simulink model "LateralControlTutorial"  (R2021a)
settings: Solver=ode1  StartTime=0.0  StopTime=simStopTime  FixedStep=1e-3  MaxStep=1e-2  MinStep=1e-3  RelTol=5e-3
PostLoadFcn:
  | addpath(fullfile(matlabroot,'toolbox','shared','drivingscenario'));
  | helperLateralControlTutorialSetup
values from neighbouring files (symbols this model uses):
  directions = ones(size(refPoses, 1), 1)    [helperLateralControlTutorialSetup.m]
  speed = 10    [helperCreateDrivingScenario.m]
  speedProfile = ones(size(refPoses, 1), 1)*speed    [helperLateralControlTutorialSetup.m]
  Ts = 0.05    [helperLateralControlTutorialSetup.m]
  wheelbase = 2.8    [helperLateralControlTutorialSetup.m]
undefined symbols (not defined in the file or in its folder): curvatures, refPoses, theta0, x0, y0
libraries: pid_lib x6, simulink_extras x3, drivingvehiclecontroller x2, dspstat3 x1, drivingscenarioandsensors x1, autolibshared x1
settings Model: PacingRate=0.750000  Creator=The MathWorks, Inc.  LastModifiedBy=efrem
settings SolverCC: ZeroCrossAlgorithm=Adaptive  AlgebraicLoopSolver=TrustRegion  DecoupledContinuousIntegration=on  MinimalZcImpactIntegration=on
settings DataIOCC: DSMLogging=off  ReturnWorkspaceOutputs=off
settings DebuggingCC: SFMachineParentedDataDiag=warning  UnderSpecifiedDimensionMsg=warning  ArithmeticOperatorsInVariantConditions=warning
settings SFSimCC: SimUseLocalCustomCode=off  CustomCodeUndefinedFunction=UseInterfaceOnly
settings RTWCC: RTWUseLocalCustomCode=off

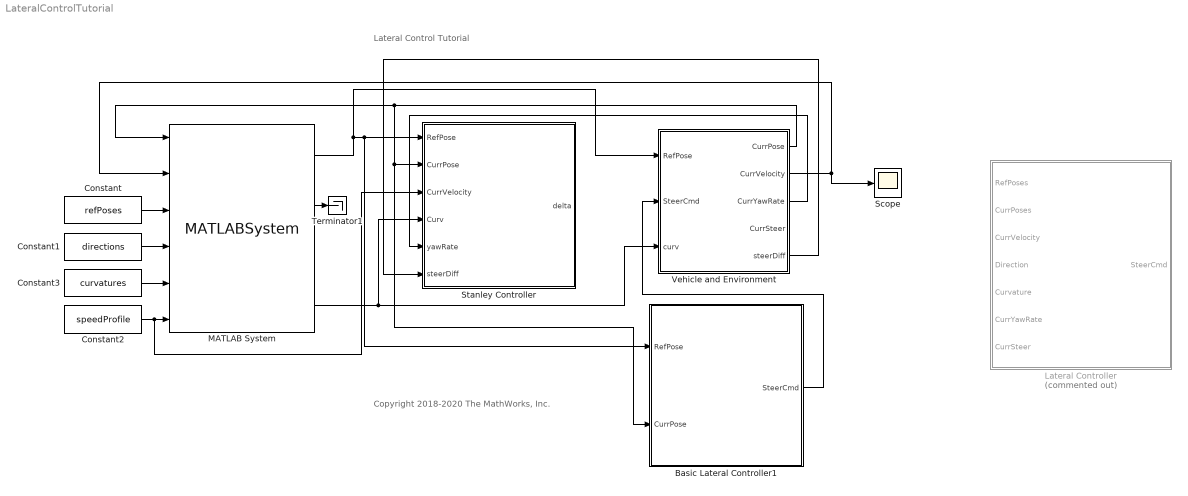
== system LateralControlTutorial ==
  note: Lateral Control Tutorial
  note: Copyright 2018-2020 The MathWorks, Inc.
  Basic Lateral Controller1 : Subsystem
  Constant : Constant  Value=refPoses
  Constant1 : Constant  Value=directions
  Constant2 : Constant  Value=speedProfile
  Constant3 : Constant  Value=curvatures
  Lateral Controller : Subsystem  Commented=on  Variant=on  VariantControlMode=label  VariantControl=Kinematic  LabelModeActiveChoice=Dynamic
  MATLAB System : MATLABSystem  System=HelperPathAnalyzer  Wheelbase=2.8  HasResetOutput=off  SimulateUsing=Interpreted execution
      mask Type: HelperPathAnalyzer
      mask Display:
      | disp(['Helper' char(10) 'Path' char(10) 'Analyzer']);
      | port_label('input',1,'CurrPose');
      | port_label('input',2,'CurrVelocity');
      | port_label('input',3,'RefPoses');
      | port_label('input',4,'Directions');
      | port_label('input',5,'Curvatures');
      | port_label('input',6,'RefVelocities');
      | port_label('output',1,'RefPose');
      | port_label('output',2,'RefVelocity');
      | port_label('output',3,'Direction');
      | port_label('output',4,'Curvature');
  Scope : Scope
  Stanley Controller : Subsystem
  Terminator1 : Terminator
  Vehicle and Environment : Subsystem
  wires:
  Constant/1 -> MATLAB System/3
  MATLAB System/2 -> Terminator1/1
  Constant1/1 -> MATLAB System/4
  Vehicle and Environment/1(CurrPose) -> Basic Lateral Controller1/2(CurrPose), Stanley Controller/2(CurrPose), MATLAB System/1
  Vehicle and Environment/2(CurrVelocity) -> Scope/1, MATLAB System/2
  MATLAB System/1 -> Basic Lateral Controller1/1(RefPose), Stanley Controller/1(RefPose), Vehicle and Environment/1(RefPose)
  MATLAB System/4 -> Stanley Controller/4(Curv), Vehicle and Environment/3(curv)
  Constant3/1 -> MATLAB System/5
  Constant2/1 -> Stanley Controller/3(CurrVelocity), MATLAB System/6
  Basic Lateral Controller1/1(SteerCmd) -> Vehicle and Environment/2(SteerCmd)
  Vehicle and Environment/3(CurrYawRate) -> Stanley Controller/5(yawRate)
  Vehicle and Environment/5(steerDiff) -> Stanley Controller/6(steerDiff)

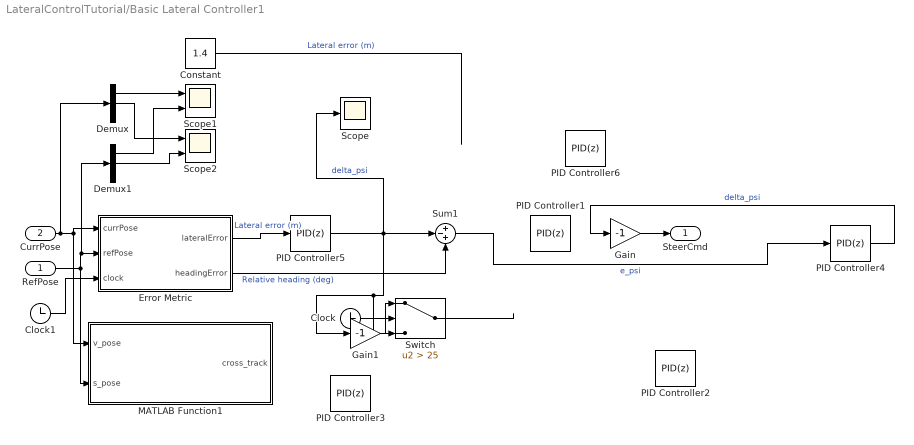
== system LateralControlTutorial/Basic Lateral Controller1 ==
  RefPose : Inport
  CurrPose : Inport  Port=2
  Clock : Clock
  Clock1 : Clock
  Constant : Constant  Value=1.4
  Demux : Demux  Outputs=3
  Demux1 : Demux  Outputs=3
  Error Metric : MATLAB Function  TreatAsAtomicUnit=on  mask{wheelbase=wheelbase}
      mask prompts: wheelbase "Wheelbase of vehicle"
  Gain : Gain  Gain=-1
  Gain1 : Gain  Gain=-1
  MATLAB Function1 : MATLAB Function  TreatAsAtomicUnit=on
  PID Controller1 : pid_lib/PID Controller  Controller=PID  Form=Parallel  TimeDomain=Discrete-time  UseExternalTs=off  SampleTime=-1  IntegratorMethod=Forward Euler  FilterMethod=Forward Euler  ControllerParametersSource=internal  P=0.67  I=0.12  D=0.32  UseFilter=on  N=100  TunerSelectOption=Transfer Function Based (PID Tuner App)  InitialConditionSource=internal  InitialConditionForIntegrator=0  InitialConditionForFilter=0  DifferentiatorICPrevScaledInput=0  ExternalReset=none  TrackingMode=off  Kt=1  LimitOutput=on  SatLimitsSource=internal  UpperSaturationLimit=45  LowerSaturationLimit=-45  LinearizeAsGain=on  AntiWindupMode=none  Kb=1  POutMin=[]  POutMax=[]  IOutMin=[]  IOutMax=[]  DOutMin=[]  DOutMax=[]  NOutMin=[]  NOutMax=[]  SumOutMin=[]  SumOutMax=[]  SaturationOutMin=[]  SaturationOutMax=[]  PParamMin=[]  PParamMax=[]  IParamMin=[]  IParamMax=[]  DParamMin=[]  DParamMax=[]  NParamMin=[]  NParamMax=[]  KbParamMin=[]  KbParamMax=[]  KtParamMin=[]  KtParamMax=[]  KbOutMin=[]  KbOutMax=[]  KtOutMin=[]  KtOutMax=[]  IntegratorOutMin=[]  IntegratorOutMax=[]  FilterOutMin=[]  FilterOutMax=[]  SumI1OutMin=[]  SumI1OutMax=[]  SumI2OutMin=[]  SumI2OutMax=[]  SumI3OutMin=[]  SumI3OutMax=[]  SumI4OutMin=[]  SumI4OutMax=[]  SumDOutMin=[]  SumDOutMax=[]  DifferentiatorOutMin=[]  DifferentiatorOutMax=[]  FilterDiffOutCoefMin=[]  FilterDiffOutCoefMax=[]  ReciprocalOutMin=[]  ReciprocalOutMax=[]  SumDenOutMin=[]  SumDenOutMax=[]  SumNumOutMin=[]  SumNumOutMax=[]  DivideOutMin=[]  DivideOutMax=[]  UdiffTsProdOutMin=[]  UdiffTsProdOutMax=[]  NTsProdOutMin=[]  NTsProdOutMax=[]  UintegralTsProdOutMin=[]  UintegralTsProdOutMax=[]  UngainTsProdOutMin=[]  UngainTsProdOutMax=[]  IntegratorContinuousStateAttributes=''  IntegratorStateMustResolveToSignalObject=off  IntegratorRTWStateStorageClass=Auto  FilterContinuousStateAttributes=''  FilterStateMustResolveToSignalObject=off  FilterRTWStateStorageClass=Auto  ParallelPVariant=InternalParameters  IdealPVariant=Disabled  IVariant=InternalParameters  DVariant=InternalParameters  IntegratorVariant=Discrete  SatVariant=Enabled  AWVariant=Passthrough  PCopyVariant=Disabled  TRVariant=Disabled  FdbkBlocksVariant=Forward  IdealPFdbkVariant=Disabled  SatFdbkVariant=Disabled  DerivativeFilterVariant=ForwardEulerFilter  NVariant=InternalParameters  NCopyVariant=Disabled  FilterICVariant=InternalICsFilter  IntegratorICVariant=InternalICs  ExternalResetVariant=Disabled  TRSumVariant=Passthrough  SumFdbkVariant=Disabled  SumVariant=Sum_PID  TsampFilterVariant=InternalTs  TsampNgainVariant=Passthrough  TsampIntegralVariant=Passthrough  ExternalSaturationOutDataTypeStr=Inherit: Same as second input
  PID Controller2 : pid_lib/PID Controller  Controller=PID  Form=Parallel  TimeDomain=Discrete-time  UseExternalTs=off  SampleTime=-1  IntegratorMethod=Forward Euler  FilterMethod=Forward Euler  ControllerParametersSource=internal  P=1.5  I=0.4  D=0.4  UseFilter=on  N=1000  TunerSelectOption=Transfer Function Based (PID Tuner App)  InitialConditionSource=internal  InitialConditionForIntegrator=0  InitialConditionForFilter=0  DifferentiatorICPrevScaledInput=0  ExternalReset=none  TrackingMode=off  Kt=1  LimitOutput=on  SatLimitsSource=internal  UpperSaturationLimit=45  LowerSaturationLimit=-45  LinearizeAsGain=on  AntiWindupMode=none  Kb=1  POutMin=[]  POutMax=[]  IOutMin=[]  IOutMax=[]  DOutMin=[]  DOutMax=[]  NOutMin=[]  NOutMax=[]  SumOutMin=[]  SumOutMax=[]  SaturationOutMin=[]  SaturationOutMax=[]  PParamMin=[]  PParamMax=[]  IParamMin=[]  IParamMax=[]  DParamMin=[]  DParamMax=[]  NParamMin=[]  NParamMax=[]  KbParamMin=[]  KbParamMax=[]  KtParamMin=[]  KtParamMax=[]  KbOutMin=[]  KbOutMax=[]  KtOutMin=[]  KtOutMax=[]  IntegratorOutMin=[]  IntegratorOutMax=[]  FilterOutMin=[]  FilterOutMax=[]  SumI1OutMin=[]  SumI1OutMax=[]  SumI2OutMin=[]  SumI2OutMax=[]  SumI3OutMin=[]  SumI3OutMax=[]  SumI4OutMin=[]  SumI4OutMax=[]  SumDOutMin=[]  SumDOutMax=[]  DifferentiatorOutMin=[]  DifferentiatorOutMax=[]  FilterDiffOutCoefMin=[]  FilterDiffOutCoefMax=[]  ReciprocalOutMin=[]  ReciprocalOutMax=[]  SumDenOutMin=[]  SumDenOutMax=[]  SumNumOutMin=[]  SumNumOutMax=[]  DivideOutMin=[]  DivideOutMax=[]  UdiffTsProdOutMin=[]  UdiffTsProdOutMax=[]  NTsProdOutMin=[]  NTsProdOutMax=[]  UintegralTsProdOutMin=[]  UintegralTsProdOutMax=[]  UngainTsProdOutMin=[]  UngainTsProdOutMax=[]  IntegratorContinuousStateAttributes=''  IntegratorStateMustResolveToSignalObject=off  IntegratorRTWStateStorageClass=Auto  FilterContinuousStateAttributes=''  FilterStateMustResolveToSignalObject=off  FilterRTWStateStorageClass=Auto  ParallelPVariant=InternalParameters  IdealPVariant=Disabled  IVariant=InternalParameters  DVariant=InternalParameters  IntegratorVariant=Discrete  SatVariant=Enabled  AWVariant=Passthrough  PCopyVariant=Disabled  TRVariant=Disabled  FdbkBlocksVariant=Forward  IdealPFdbkVariant=Disabled  SatFdbkVariant=Disabled  DerivativeFilterVariant=ForwardEulerFilter  NVariant=InternalParameters  NCopyVariant=Disabled  FilterICVariant=InternalICsFilter  IntegratorICVariant=InternalICs  ExternalResetVariant=Disabled  TRSumVariant=Passthrough  SumFdbkVariant=Disabled  SumVariant=Sum_PID  TsampFilterVariant=InternalTs  TsampNgainVariant=Passthrough  TsampIntegralVariant=Passthrough  ExternalSaturationOutDataTypeStr=Inherit: Same as second input
  PID Controller3 : pid_lib/PID Controller  Controller=PID  Form=Parallel  TimeDomain=Discrete-time  UseExternalTs=off  SampleTime=-1  IntegratorMethod=Forward Euler  FilterMethod=Forward Euler  ControllerParametersSource=internal  P=0.4  I=0  D=0  UseFilter=on  N=100  TunerSelectOption=Transfer Function Based (PID Tuner App)  InitialConditionSource=internal  InitialConditionForIntegrator=0  InitialConditionForFilter=0  DifferentiatorICPrevScaledInput=0  ExternalReset=none  TrackingMode=off  Kt=1  LimitOutput=off  SatLimitsSource=internal  UpperSaturationLimit=0.5  LowerSaturationLimit=-0.5  LinearizeAsGain=on  AntiWindupMode=none  Kb=1  POutMin=[]  POutMax=[]  IOutMin=[]  IOutMax=[]  DOutMin=[]  DOutMax=[]  NOutMin=[]  NOutMax=[]  SumOutMin=[]  SumOutMax=[]  SaturationOutMin=[]  SaturationOutMax=[]  PParamMin=[]  PParamMax=[]  IParamMin=[]  IParamMax=[]  DParamMin=[]  DParamMax=[]  NParamMin=[]  NParamMax=[]  KbParamMin=[]  KbParamMax=[]  KtParamMin=[]  KtParamMax=[]  KbOutMin=[]  KbOutMax=[]  KtOutMin=[]  KtOutMax=[]  IntegratorOutMin=[]  IntegratorOutMax=[]  FilterOutMin=[]  FilterOutMax=[]  SumI1OutMin=[]  SumI1OutMax=[]  SumI2OutMin=[]  SumI2OutMax=[]  SumI3OutMin=[]  SumI3OutMax=[]  SumI4OutMin=[]  SumI4OutMax=[]  SumDOutMin=[]  SumDOutMax=[]  DifferentiatorOutMin=[]  DifferentiatorOutMax=[]  FilterDiffOutCoefMin=[]  FilterDiffOutCoefMax=[]  ReciprocalOutMin=[]  ReciprocalOutMax=[]  SumDenOutMin=[]  SumDenOutMax=[]  SumNumOutMin=[]  SumNumOutMax=[]  DivideOutMin=[]  DivideOutMax=[]  UdiffTsProdOutMin=[]  UdiffTsProdOutMax=[]  NTsProdOutMin=[]  NTsProdOutMax=[]  UintegralTsProdOutMin=[]  UintegralTsProdOutMax=[]  UngainTsProdOutMin=[]  UngainTsProdOutMax=[]  IntegratorContinuousStateAttributes=''  IntegratorStateMustResolveToSignalObject=off  IntegratorRTWStateStorageClass=Auto  FilterContinuousStateAttributes=''  FilterStateMustResolveToSignalObject=off  FilterRTWStateStorageClass=Auto  ParallelPVariant=InternalParameters  IdealPVariant=Disabled  IVariant=InternalParameters  DVariant=InternalParameters  IntegratorVariant=Discrete  SatVariant=Disabled  AWVariant=Passthrough  PCopyVariant=Disabled  TRVariant=Disabled  FdbkBlocksVariant=Forward  IdealPFdbkVariant=Disabled  SatFdbkVariant=Disabled  DerivativeFilterVariant=ForwardEulerFilter  NVariant=InternalParameters  NCopyVariant=Disabled  FilterICVariant=InternalICsFilter  IntegratorICVariant=InternalICs  ExternalResetVariant=Disabled  TRSumVariant=Passthrough  SumFdbkVariant=Disabled  SumVariant=Sum_PID  TsampFilterVariant=InternalTs  TsampNgainVariant=Passthrough  TsampIntegralVariant=Passthrough  ExternalSaturationOutDataTypeStr=Inherit: Same as second input
  PID Controller4 : pid_lib/PID Controller  Controller=PID  Form=Parallel  TimeDomain=Discrete-time  UseExternalTs=off  SampleTime=-1  IntegratorMethod=Forward Euler  FilterMethod=Forward Euler  ControllerParametersSource=internal  P=1.5  I=0.4  D=0.4  UseFilter=on  N=600  TunerSelectOption=Transfer Function Based (PID Tuner App)  InitialConditionSource=internal  InitialConditionForIntegrator=0  InitialConditionForFilter=0  DifferentiatorICPrevScaledInput=0  ExternalReset=none  TrackingMode=off  Kt=1  LimitOutput=on  SatLimitsSource=internal  UpperSaturationLimit=45  LowerSaturationLimit=-45  LinearizeAsGain=on  AntiWindupMode=none  Kb=1  POutMin=[]  POutMax=[]  IOutMin=[]  IOutMax=[]  DOutMin=[]  DOutMax=[]  NOutMin=[]  NOutMax=[]  SumOutMin=[]  SumOutMax=[]  SaturationOutMin=[]  SaturationOutMax=[]  PParamMin=[]  PParamMax=[]  IParamMin=[]  IParamMax=[]  DParamMin=[]  DParamMax=[]  NParamMin=[]  NParamMax=[]  KbParamMin=[]  KbParamMax=[]  KtParamMin=[]  KtParamMax=[]  KbOutMin=[]  KbOutMax=[]  KtOutMin=[]  KtOutMax=[]  IntegratorOutMin=[]  IntegratorOutMax=[]  FilterOutMin=[]  FilterOutMax=[]  SumI1OutMin=[]  SumI1OutMax=[]  SumI2OutMin=[]  SumI2OutMax=[]  SumI3OutMin=[]  SumI3OutMax=[]  SumI4OutMin=[]  SumI4OutMax=[]  SumDOutMin=[]  SumDOutMax=[]  DifferentiatorOutMin=[]  DifferentiatorOutMax=[]  FilterDiffOutCoefMin=[]  FilterDiffOutCoefMax=[]  ReciprocalOutMin=[]  ReciprocalOutMax=[]  SumDenOutMin=[]  SumDenOutMax=[]  SumNumOutMin=[]  SumNumOutMax=[]  DivideOutMin=[]  DivideOutMax=[]  UdiffTsProdOutMin=[]  UdiffTsProdOutMax=[]  NTsProdOutMin=[]  NTsProdOutMax=[]  UintegralTsProdOutMin=[]  UintegralTsProdOutMax=[]  UngainTsProdOutMin=[]  UngainTsProdOutMax=[]  IntegratorContinuousStateAttributes=''  IntegratorStateMustResolveToSignalObject=off  IntegratorRTWStateStorageClass=Auto  FilterContinuousStateAttributes=''  FilterStateMustResolveToSignalObject=off  FilterRTWStateStorageClass=Auto  ParallelPVariant=InternalParameters  IdealPVariant=Disabled  IVariant=InternalParameters  DVariant=InternalParameters  IntegratorVariant=Discrete  SatVariant=Enabled  AWVariant=Passthrough  PCopyVariant=Disabled  TRVariant=Disabled  FdbkBlocksVariant=Forward  IdealPFdbkVariant=Disabled  SatFdbkVariant=Disabled  DerivativeFilterVariant=ForwardEulerFilter  NVariant=InternalParameters  NCopyVariant=Disabled  FilterICVariant=InternalICsFilter  IntegratorICVariant=InternalICs  ExternalResetVariant=Disabled  TRSumVariant=Passthrough  SumFdbkVariant=Disabled  SumVariant=Sum_PID  TsampFilterVariant=InternalTs  TsampNgainVariant=Passthrough  TsampIntegralVariant=Passthrough  ExternalSaturationOutDataTypeStr=Inherit: Same as second input
  PID Controller5 : pid_lib/PID Controller  Controller=PID  Form=Parallel  TimeDomain=Discrete-time  UseExternalTs=off  SampleTime=-1  IntegratorMethod=Forward Euler  FilterMethod=Forward Euler  ControllerParametersSource=internal  P=8  I=2  D=0  UseFilter=on  N=100  TunerSelectOption=Transfer Function Based (PID Tuner App)  InitialConditionSource=internal  InitialConditionForIntegrator=0  InitialConditionForFilter=0  DifferentiatorICPrevScaledInput=0  ExternalReset=none  TrackingMode=off  Kt=1  LimitOutput=off  SatLimitsSource=internal  UpperSaturationLimit=0.5  LowerSaturationLimit=-0.5  LinearizeAsGain=on  AntiWindupMode=none  Kb=1  POutMin=[]  POutMax=[]  IOutMin=[]  IOutMax=[]  DOutMin=[]  DOutMax=[]  NOutMin=[]  NOutMax=[]  SumOutMin=[]  SumOutMax=[]  SaturationOutMin=[]  SaturationOutMax=[]  PParamMin=[]  PParamMax=[]  IParamMin=[]  IParamMax=[]  DParamMin=[]  DParamMax=[]  NParamMin=[]  NParamMax=[]  KbParamMin=[]  KbParamMax=[]  KtParamMin=[]  KtParamMax=[]  KbOutMin=[]  KbOutMax=[]  KtOutMin=[]  KtOutMax=[]  IntegratorOutMin=[]  IntegratorOutMax=[]  FilterOutMin=[]  FilterOutMax=[]  SumI1OutMin=[]  SumI1OutMax=[]  SumI2OutMin=[]  SumI2OutMax=[]  SumI3OutMin=[]  SumI3OutMax=[]  SumI4OutMin=[]  SumI4OutMax=[]  SumDOutMin=[]  SumDOutMax=[]  DifferentiatorOutMin=[]  DifferentiatorOutMax=[]  FilterDiffOutCoefMin=[]  FilterDiffOutCoefMax=[]  ReciprocalOutMin=[]  ReciprocalOutMax=[]  SumDenOutMin=[]  SumDenOutMax=[]  SumNumOutMin=[]  SumNumOutMax=[]  DivideOutMin=[]  DivideOutMax=[]  UdiffTsProdOutMin=[]  UdiffTsProdOutMax=[]  NTsProdOutMin=[]  NTsProdOutMax=[]  UintegralTsProdOutMin=[]  UintegralTsProdOutMax=[]  UngainTsProdOutMin=[]  UngainTsProdOutMax=[]  IntegratorContinuousStateAttributes=''  IntegratorStateMustResolveToSignalObject=off  IntegratorRTWStateStorageClass=Auto  FilterContinuousStateAttributes=''  FilterStateMustResolveToSignalObject=off  FilterRTWStateStorageClass=Auto  ParallelPVariant=InternalParameters  IdealPVariant=Disabled  IVariant=InternalParameters  DVariant=InternalParameters  IntegratorVariant=Discrete  SatVariant=Disabled  AWVariant=Passthrough  PCopyVariant=Disabled  TRVariant=Disabled  FdbkBlocksVariant=Forward  IdealPFdbkVariant=Disabled  SatFdbkVariant=Disabled  DerivativeFilterVariant=ForwardEulerFilter  NVariant=InternalParameters  NCopyVariant=Disabled  FilterICVariant=InternalICsFilter  IntegratorICVariant=InternalICs  ExternalResetVariant=Disabled  TRSumVariant=Passthrough  SumFdbkVariant=Disabled  SumVariant=Sum_PID  TsampFilterVariant=InternalTs  TsampNgainVariant=Passthrough  TsampIntegralVariant=Passthrough  ExternalSaturationOutDataTypeStr=Inherit: Same as second input
  PID Controller6 : pid_lib/PID Controller  Controller=PID  Form=Parallel  TimeDomain=Discrete-time  UseExternalTs=off  SampleTime=-1  IntegratorMethod=Forward Euler  FilterMethod=Forward Euler  ControllerParametersSource=internal  P=2  I=0.02  D=0  UseFilter=on  N=100  TunerSelectOption=Transfer Function Based (PID Tuner App)  InitialConditionSource=internal  InitialConditionForIntegrator=0  InitialConditionForFilter=0  DifferentiatorICPrevScaledInput=0  ExternalReset=none  TrackingMode=off  Kt=1  LimitOutput=off  SatLimitsSource=internal  UpperSaturationLimit=0.5  LowerSaturationLimit=-0.5  LinearizeAsGain=on  AntiWindupMode=none  Kb=1  POutMin=[]  POutMax=[]  IOutMin=[]  IOutMax=[]  DOutMin=[]  DOutMax=[]  NOutMin=[]  NOutMax=[]  SumOutMin=[]  SumOutMax=[]  SaturationOutMin=[]  SaturationOutMax=[]  PParamMin=[]  PParamMax=[]  IParamMin=[]  IParamMax=[]  DParamMin=[]  DParamMax=[]  NParamMin=[]  NParamMax=[]  KbParamMin=[]  KbParamMax=[]  KtParamMin=[]  KtParamMax=[]  KbOutMin=[]  KbOutMax=[]  KtOutMin=[]  KtOutMax=[]  IntegratorOutMin=[]  IntegratorOutMax=[]  FilterOutMin=[]  FilterOutMax=[]  SumI1OutMin=[]  SumI1OutMax=[]  SumI2OutMin=[]  SumI2OutMax=[]  SumI3OutMin=[]  SumI3OutMax=[]  SumI4OutMin=[]  SumI4OutMax=[]  SumDOutMin=[]  SumDOutMax=[]  DifferentiatorOutMin=[]  DifferentiatorOutMax=[]  FilterDiffOutCoefMin=[]  FilterDiffOutCoefMax=[]  ReciprocalOutMin=[]  ReciprocalOutMax=[]  SumDenOutMin=[]  SumDenOutMax=[]  SumNumOutMin=[]  SumNumOutMax=[]  DivideOutMin=[]  DivideOutMax=[]  UdiffTsProdOutMin=[]  UdiffTsProdOutMax=[]  NTsProdOutMin=[]  NTsProdOutMax=[]  UintegralTsProdOutMin=[]  UintegralTsProdOutMax=[]  UngainTsProdOutMin=[]  UngainTsProdOutMax=[]  IntegratorContinuousStateAttributes=''  IntegratorStateMustResolveToSignalObject=off  IntegratorRTWStateStorageClass=Auto  FilterContinuousStateAttributes=''  FilterStateMustResolveToSignalObject=off  FilterRTWStateStorageClass=Auto  ParallelPVariant=InternalParameters  IdealPVariant=Disabled  IVariant=InternalParameters  DVariant=InternalParameters  IntegratorVariant=Discrete  SatVariant=Disabled  AWVariant=Passthrough  PCopyVariant=Disabled  TRVariant=Disabled  FdbkBlocksVariant=Forward  IdealPFdbkVariant=Disabled  SatFdbkVariant=Disabled  DerivativeFilterVariant=ForwardEulerFilter  NVariant=InternalParameters  NCopyVariant=Disabled  FilterICVariant=InternalICsFilter  IntegratorICVariant=InternalICs  ExternalResetVariant=Disabled  TRSumVariant=Passthrough  SumFdbkVariant=Disabled  SumVariant=Sum_PID  TsampFilterVariant=InternalTs  TsampNgainVariant=Passthrough  TsampIntegralVariant=Passthrough  ExternalSaturationOutDataTypeStr=Inherit: Same as second input
  Scope : Scope
  Scope1 : Scope  NumInputPorts=2
  Scope2 : Scope  NumInputPorts=2
  Sum1 : Sum  Inputs=+-+
  Switch : Switch  Criteria=u2 > Threshold  Threshold=25
  SteerCmd : Outport
  wires:
  PID Controller5/1 -> Sum1/2, Switch/3, Gain1/1, Scope/1  "delta_psi"
  Sum1/1 -> PID Controller4/1  "e_psi"
  PID Controller4/1 -> Gain/1  "delta_psi"
  CurrPose/1 -> Demux/1, MATLAB Function1/1(v_pose), Error Metric/1(currPose)
  RefPose/1 -> MATLAB Function1/2(s_pose), Demux1/1, Error Metric/2(refPose)
  Error Metric/1(lateralError) -> PID Controller5/1  "Lateral error (m)"
  Error Metric/2(headingError) -> Sum1/3  "Relative heading (deg)"
  Gain/1 -> SteerCmd/1
  Constant/1 -> ?  "Lateral error (m)"
  Clock/1 -> Switch/2
  Gain1/1 -> Switch/1
  Clock1/1 -> Error Metric/3(clock)
  Demux/1 -> Scope1/1
  Demux1/1 -> Scope1/2
  Demux/2 -> Scope2/1
  Demux1/2 -> Scope2/2
  Switch/1 -> ?

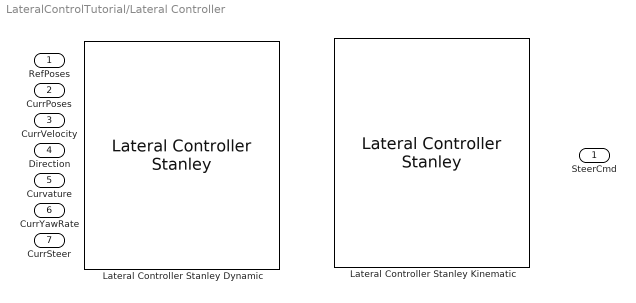
== system LateralControlTutorial/Lateral Controller ==
  "RefPoses " : Inport
  "CurrPoses " : Inport  Port=2
  "CurrVelocity " : Inport  Port=3
  "Direction " : Inport  Port=4
  "Curvature " : Inport  Port=5
  "CurrYawRate " : Inport  Port=6
  "CurrSteer " : Inport  Port=7
  Lateral Controller Stanley Dynamic : drivingvehiclecontroller/Lateral Controller Stanley  VariantControl=Dynamic  ModelType=Dynamic bicycle model  PositionGainF=2.5  PositionGainR=2.5  YawRateGain=0.5  DelayGain=0.2  VehicleMass=1575  Lf=1.2  Lr=1.6  TireStiffness=19000  Wheelbase=wheelbase  MaxSteeringAngle=35
      settings: SourceProductBaseCode=DR
  Lateral Controller Stanley Kinematic : drivingvehiclecontroller/Lateral Controller Stanley  VariantControl=Kinematic  ModelType=Kinematic bicycle model  PositionGainF=2.5  PositionGainR=2.5  YawRateGain=0.2  DelayGain=0.2  VehicleMass=1575  Lf=1.2  Lr=1.6  TireStiffness=19000  Wheelbase=wheelbase  MaxSteeringAngle=35
      settings: SourceProductBaseCode=DR
  " SteerCmd" : Outport  VectorParamsAs1DForOutWhenUnconnected=off

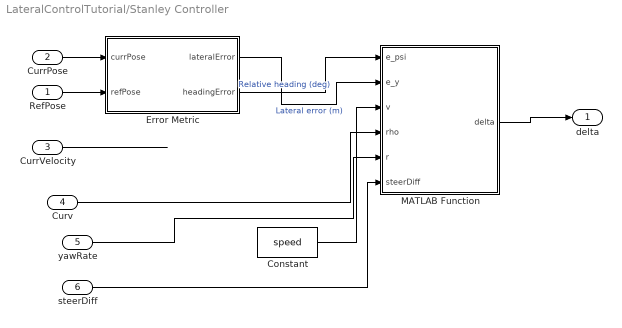
== system LateralControlTutorial/Stanley Controller ==
  RefPose : Inport
  CurrPose : Inport  Port=2
  CurrVelocity : Inport  Port=3
  Curv : Inport  Port=4
  yawRate : Inport  Port=5
  steerDiff : Inport  Port=6
  Constant : Constant  Value=speed
  Error Metric : MATLAB Function  TreatAsAtomicUnit=on  mask{wheelbase=wheelbase}
      mask prompts: wheelbase "Wheelbase of vehicle"
  MATLAB Function : MATLAB Function  TreatAsAtomicUnit=on
  delta : Outport
  wires:
  CurrPose/1 -> Error Metric/1(currPose)
  RefPose/1 -> Error Metric/2(refPose)
  Error Metric/1(lateralError) -> MATLAB Function/2(e_y)  "Lateral error (m)"
  Error Metric/2(headingError) -> MATLAB Function/1(e_psi)  "Relative heading (deg)"
  CurrVelocity/1 -> ?
  Curv/1 -> MATLAB Function/4(rho)
  yawRate/1 -> MATLAB Function/5(r)
  MATLAB Function/1(delta) -> delta/1
  Constant/1 -> MATLAB Function/3(v)
  steerDiff/1 -> MATLAB Function/6(steerDiff)

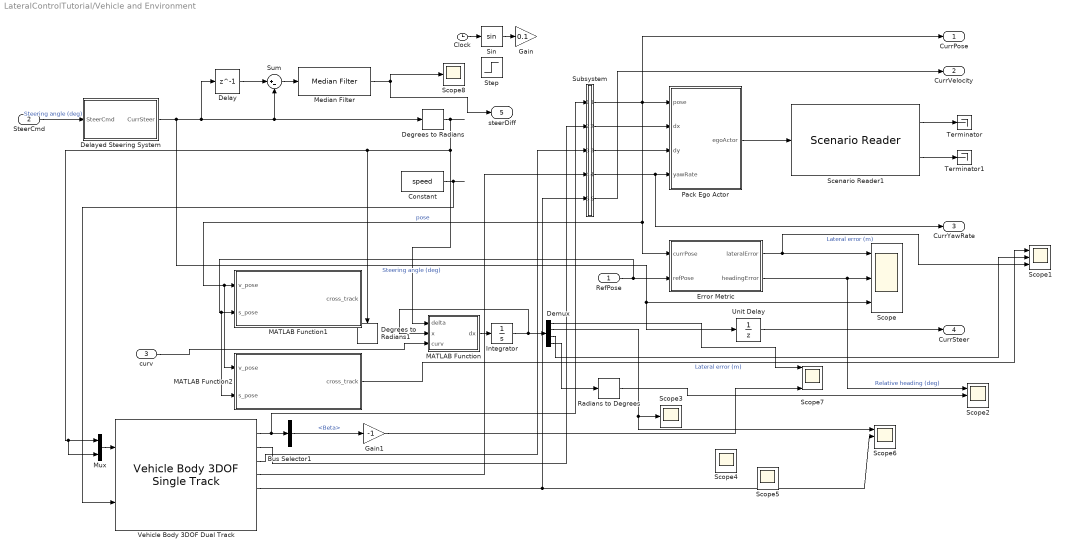
== system LateralControlTutorial/Vehicle and Environment ==
  RefPose : Inport
  SteerCmd : Inport  Port=2
  curv : Inport  Port=3
  Bus Selector1 : BusSelector  OutputSignals=BdyFrm.Cg.Ang.Beta
  Clock : Clock
  Constant : Constant  Value=speed
  Degrees to Radians : simulink_extras/Transformations/Degrees to Radians
  Degrees to Radians1 : simulink_extras/Transformations/Degrees to Radians
  Delay : Delay  DelayLength=1
  Delayed Steering System : Subsystem
  Demux : Demux
  Error Metric : MATLAB Function  TreatAsAtomicUnit=on  mask{wheelbase=wheelbase}
      mask prompts: wheelbase "Wheelbase of vehicle"
  Gain : Gain  Gain=0.1
  Gain1 : Gain  Gain=-1
  Integrator : Integrator  InitialCondition=[0; 0;0;0]
  MATLAB Function : MATLAB Function  TreatAsAtomicUnit=on
  MATLAB Function1 : MATLAB Function  TreatAsAtomicUnit=on
  MATLAB Function2 : MATLAB Function  TreatAsAtomicUnit=on
  Median Filter : dspstat3/Median Filter  WindowLength=10  SimulateUsing=Interpreted execution
      settings: SourceProductBaseCode=DS
  Mux : Mux  Inputs=2
  Pack Ego Actor : MATLAB Function  TreatAsAtomicUnit=on
  Radians to Degrees : simulink_extras/Transformations/Radians to Degrees
  Scenario Reader1 : drivingscenarioandsensors/Scenario Reader  ScenarioSource=From file  ScenarioFileName=LateralControl.mat  ScenarioVariableName=scenario  OutputCoordinateSystem=Vehicle coordinates  EgoVehicleSource=Input port  EgoVehicleActorID=1  OrientVehiclesOnRoad=off  OutputEgoVehiclePose=off  SampleTime=Ts  LaneBoundaryOutput=Ego vehicle lane boundaries  LaneBoundaryDistance=0:0.5:9.5  LaneBoundaryLocation=Center of lane markings  BusNameSource=Property  BusName=BusActors  BusNumActorsSource=Scenario  BusNumActors=100  BusName2Source=Auto  BusName2=BusLaneBoundaries  BusNumLaneBoundariesSource=Scenario  BusNumLaneBoundaries=10  BusName3Source=Auto  BusName3=BusEgoActor  ShowCoordinateLabels=on  SimulateUsing=Interpreted execution
  Scope{,1..2,6} (4 alike) : Scope  NumInputPorts=3
  Scope{3..5,8} (4 alike) : Scope
  Scope7 : Scope  NumInputPorts=4
  Sin : Trigonometry
  Step : Step  Time=0  After=-0.2  SampleTime=0
  Subsystem : Subsystem
  Sum : Sum  Inputs=|+-
  Terminator : Terminator
  Terminator1 : Terminator
  Unit Delay : UnitDelay  SampleTime=0.05  HasFrameUpgradeWarning=on
  Vehicle Body 3DOF Dual Track : autolibshared/Vehicle Body 3DOF Single Track  trackMode=Dual  inputMode=External longitudinal velocity  frontSteerMode=on  rearSteerMode=off  windMode=off  muMode=off  extFMode=off  extMMode=off  htchFMode=off  htchMMode=off  extXo=off  extpsio=off  extxdoto=off  extro=off  extYo=off  extTamb=off  extydoto=off  aMode=2  NF=2  NR=2  m=2000  a=1.4  b=1.6  h=0.35  dh=1  hh=0.2  X_o=0  xdot_o=0  CalphaMode=off  sigmaMode=on  d=0  hl=0  w=[1.4,1.4]  Cy_f=12e3  Cy_r=11e3  sigma_f=.1  sigma_r=.1  alpha_f_brk=[-.1 .1]  Cy_f_data=[-9e3 9e3]  alpha_r_brk=[-.1 .1]  Cy_r_data=[-9e3 9e3]  Y_o=0  ydot_o=0  Izz=4000  psi_o=0  r_o=0  Af=2  Cd=.3  Cl=.1  Cpm=.1  beta_w=[0:0.01:0.3]  Cs=[0:0.03:0.9]  Cym=[0:0.01:0.3]  Pabs=101325  Tair=273  g=9.81  mu=1  xdot_tol=.01  Fznom=5000  Fxtire_sat=7e4  Fytire_sat=7e4  longOff=0  latOff=0  vertOff=0  wrapAng=off
      settings: SourceProductBaseCode=PW,DR,MT,UV,VE
  CurrPose : Outport  VectorParamsAs1DForOutWhenUnconnected=off
  CurrVelocity : Outport  Port=2  VectorParamsAs1DForOutWhenUnconnected=off
  CurrYawRate : Outport  Port=3  VectorParamsAs1DForOutWhenUnconnected=off
  CurrSteer : Outport  Port=4  VectorParamsAs1DForOutWhenUnconnected=off
  steerDiff : Outport  Port=5
  wires:
  Subsystem/2(dx) -> Pack Ego Actor/2(dx)
  Subsystem/4(CurrYawRate) -> CurrYawRate/1, Pack Ego Actor/4(yawRate)
  Subsystem/3(dy) -> Pack Ego Actor/3(dy)
  Subsystem/1(CurrPose) -> CurrPose/1, Pack Ego Actor/1(pose), Error Metric/1(currPose), MATLAB Function2/1(v_pose), MATLAB Function1/1(v_pose)  "pose"
  Error Metric/1(lateralError) -> Scope1/3, Scope/1  "Lateral error (m)"
  RefPose/1 -> MATLAB Function2/2(s_pose), MATLAB Function1/2(s_pose), Error Metric/2(refPose)
  Error Metric/2(headingError) -> Scope2/1, Scope/2  "Relative heading (deg)"
  Degrees to Radians/1 -> Mux/2, Mux/1, Degrees to Radians1/1, MATLAB Function/1(delta)
  Constant/1 -> Vehicle Body 3DOF Dual Track/2
  Delayed Steering System/1(CurrSteer) -> Delay/1, Sum/2, Degrees to Radians/1, Unit Delay/1, Scope/3  "Steering angle (deg)"
  Unit Delay/1 -> CurrSteer/1
  Scenario Reader1/1 -> Terminator/1
  Subsystem/5(CurrVelocity) -> CurrVelocity/1
  Scenario Reader1/2 -> Terminator1/1
  Pack Ego Actor/1(egoActor) -> Scenario Reader1/1
  MATLAB Function/1(dx) -> Integrator/1
  Integrator/1 -> MATLAB Function/2(x), Demux/1
  Demux/3 -> Scope1/2
  Demux/4 -> Radians to Degrees/1
  Radians to Degrees/1 -> Scope2/2
  SteerCmd/1 -> Delayed Steering System/1(SteerCmd)  "Steering angle (deg)"
  MATLAB Function2/1(cross_track) -> Scope1/1  "Lateral error (m)"
  Clock/1 -> Sin/1
  Sin/1 -> Gain/1
  Demux/2 -> Scope6/1, Scope3/1
  Demux/1 -> Scope7/1
  Vehicle Body 3DOF Dual Track/5 -> Subsystem/5(In5), Scope6/2
  Vehicle Body 3DOF Dual Track/1 -> Subsystem/1(In1), Bus Selector1/1
  Bus Selector1/1 -> Gain1/1  "<Beta>"
  Mux/1 -> Vehicle Body 3DOF Dual Track/1
  Gain1/1 -> Scope7/4
  Vehicle Body 3DOF Dual Track/2 -> Subsystem/2(In2)
  Vehicle Body 3DOF Dual Track/3 -> Subsystem/3(In3)
  Vehicle Body 3DOF Dual Track/4 -> Subsystem/4(In4)
  curv/1 -> MATLAB Function/3(curv)
  Delay/1 -> Sum/1
  Sum/1 -> Median Filter/1
  Median Filter/1 -> Scope8/1, steerDiff/1

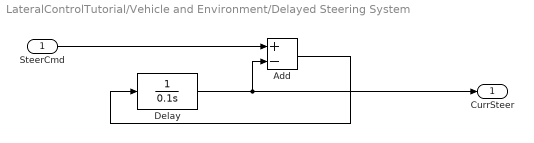
== system LateralControlTutorial/Vehicle and Environment/Delayed Steering System ==
  SteerCmd : Inport
  Add : Sum  Inputs=+-
  Delay : TransferFcn  Denominator=[0.1 0]
  CurrSteer : Outport  VectorParamsAs1DForOutWhenUnconnected=off
  wires:
  Add/1 -> Delay/1
  SteerCmd/1 -> Add/1
  Delay/1 -> CurrSteer/1, Add/2

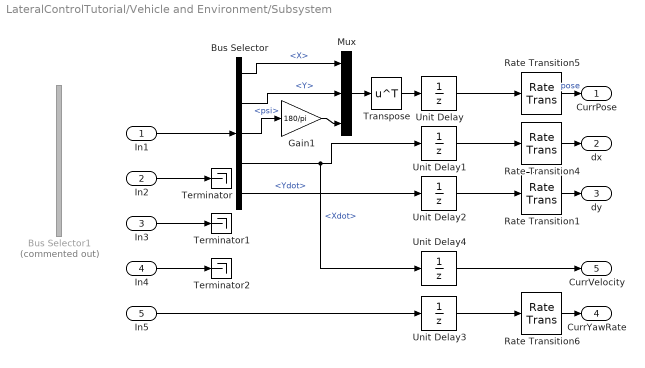
== system LateralControlTutorial/Vehicle and Environment/Subsystem ==
  In1 : Inport
  In2 : Inport  Port=2
  In3 : Inport  Port=3
  In4 : Inport  Port=4
  In5 : Inport  Port=5
  Bus Selector : BusSelector  OutputSignals=InertFrm.Cg.Disp.X,InertFrm.Cg.Disp.Y,InertFrm.Cg.Ang.psi,InertFrm.Cg.Vel.Xdot,InertFrm.Cg.Vel.Ydot
  Bus Selector1 : BusSelector  Commented=on  OutputSignals=InertFrm.RearAxl.Disp.X,InertFrm.RearAxl.Disp.Y,InertFrm.Cg.Ang.psi,InertFrm.RearAxl.Vel.Xdot,InertFrm.RearAxl.Vel.Ydot,BdyFrm.RearAxl.Vel.xdot
  Gain1 : Gain  Gain=180/pi
  Mux : Mux  Inputs=3
  Rate Transition1 : RateTransition  OutPortSampleTime=Ts
  Rate Transition4 : RateTransition  InitialCondition=speed  OutPortSampleTime=Ts
  Rate Transition5 : RateTransition  InitialCondition=[x0, y0, theta0]  OutPortSampleTime=Ts
  Rate Transition6 : RateTransition  OutPortSampleTime=Ts
  Terminator : Terminator
  Terminator1 : Terminator
  Terminator2 : Terminator
  Transpose : Math  Operator=transpose  SignedPower=on  SaturateOnIntegerOverflow=on
  Unit Delay : UnitDelay  InitialCondition=[x0, y0, theta0]  SampleTime=-1  HasFrameUpgradeWarning=on
  Unit Delay1 : UnitDelay  InitialCondition=speed  SampleTime=-1  HasFrameUpgradeWarning=on
  Unit Delay2 : UnitDelay  SampleTime=-1  HasFrameUpgradeWarning=on
  Unit Delay3 : UnitDelay  SampleTime=-1  HasFrameUpgradeWarning=on
  Unit Delay4 : UnitDelay  SampleTime=-1  HasFrameUpgradeWarning=on
  CurrPose : Outport  VectorParamsAs1DForOutWhenUnconnected=off
  dx : Outport  Port=2  VectorParamsAs1DForOutWhenUnconnected=off
  dy : Outport  Port=3  VectorParamsAs1DForOutWhenUnconnected=off
  CurrYawRate : Outport  Port=4  VectorParamsAs1DForOutWhenUnconnected=off
  CurrVelocity : Outport  Port=5  VectorParamsAs1DForOutWhenUnconnected=off
  wires:
  Bus Selector/4 -> Unit Delay4/1, Unit Delay1/1  "<Xdot>"
  Bus Selector/2 -> Mux/2  "<Y>"
  Bus Selector/1 -> Mux/1  "<X>"
  Transpose/1 -> Unit Delay/1
  Unit Delay/1 -> Rate Transition5/1
  Mux/1 -> Transpose/1
  Unit Delay3/1 -> Rate Transition6/1
  Bus Selector/5 -> Unit Delay2/1  "<Ydot>"
  Bus Selector/3 -> Gain1/1  "<psi>"
  Gain1/1 -> Mux/3
  In5/1 -> Unit Delay3/1
  In2/1 -> Terminator/1
  In1/1 -> Bus Selector/1
  In4/1 -> Terminator2/1
  Unit Delay2/1 -> Rate Transition1/1
  Unit Delay1/1 -> Rate Transition4/1
  In3/1 -> Terminator1/1
  Unit Delay4/1 -> CurrVelocity/1
  Rate Transition5/1 -> CurrPose/1  "pose"
  Rate Transition4/1 -> dx/1
  Rate Transition1/1 -> dy/1
  Rate Transition6/1 -> CurrYawRate/1

== matlab function LateralControlTutorial/Stanley Controller/Error Metric ==
  data: currPose input size=[1 3]; refPose input size=[1 3]; lateralError output; wheelbase parameter; headingError output
function [lateralError, headingError] = fcn(currPose, refPose, wheelbase)

%   Copyright 2018 The MathWorks, Inc.

currPose(:,3) = deg2rad(currPose(:,3));
refPose(:,3)  = deg2rad(refPose(:,3));

%Convert current pose to front wheel coordinate
currPoseF = coder.nullcopy(zeros(1, 3));

currPoseF = driving.internal.control.rearPoseToFrontPose(currPose, wheelbase);

lateralError = sign(refPose(2) - currPoseF(2))*norm(currPoseF(1:2) - refPose(1:2));

headingError = rad2deg(currPose(:, 3) - refPose(:,3));

== matlab function LateralControlTutorial/Vehicle and Environment/Error Metric ==
  data: currPose input size=[1 3]; refPose input size=[1 3]; lateralError output; wheelbase parameter; headingError output
function [lateralError, headingError] = fcn(currPose, refPose, wheelbase)

%   Copyright 2018 The MathWorks, Inc.

currPose(:,3) = deg2rad(currPose(:,3));
refPose(:,3)  = deg2rad(refPose(:,3));

%Convert current pose to front wheel coordinate
currPoseF = coder.nullcopy(zeros(1, 3));

currPoseF = driving.internal.control.rearPoseToFrontPose(currPose, wheelbase);

lateralError = norm(currPoseF(1:2) - refPose(1:2));

headingError = rad2deg(currPose(:, 3) - refPose(:,3));

== matlab function LateralControlTutorial/Vehicle and Environment/MATLAB Function ==
  data: delta input; dx output; x input; curv input
function dx = fcn(delta, x, curv)
% 
% cf = 1.0542e+05; %[N/rad]
% cr = 7.4705e+04; %[N/rad]
% m = 1463;  %[kg]
% v = 10;   %[m/s]
% Iz = 1968;  %[kg m2]
% lf = 0.971;  %[m]
% lr = 1.566;  %[m]


cf = 12e+03; %[N/rad]
cr = 11e+03; %[N/rad]
m = 2000;  %[kg]
v = 10;   %[m/s]
Iz = 4000;  %[kg m2]
lf = 1.4;  %[m]
lr = 1.6;  %[m]

% A = [0, 1, 0, 0;
%      0, -(cf+cr)/m/v, (cf+cr)/m, (-cf*lf+cr*lr)/m/v;
%      0, 0, 0, 1;
%      0, -(cf*lf-cr*lr)/Iz/v, (cf*lf-cr*lr)/Iz, -(cf*lf^2+cr*lr^2)/Iz/v];
% B = [0;
%     cf/m;
%     0;
%     cf*lf/Iz];

lp = lf;

A = [-(cr+cf)/m/v, (lr*cr-lf*cf)/m/v/v-1, 0, 0;
    (lr*cr-lf*cf)/Iz, -(lr^2*cr+lf^2*cf)/Iz/v, 0, 0;
    v, lp, 0, v;
    0, 1, 0, 0];
B = [cf/m;
    cf*lf/Iz;
    0;
    0];
d = [0;0;0;-v];


dx = A*x+B*delta+d*curv;

== matlab function LateralControlTutorial/Vehicle and Environment/MATLAB Function1 ==
  data: v_pose input; cross_track output; s_pose input
function cross_track = cross_track_calc(v_pose, s_pose)
    v_vec = [v_pose(1); v_pose(2)];
    s_vec = [s_pose(1); s_pose(2)];
    % vector pointing from shadow vehicle to real vehicle
    diff_vec = v_vec - s_vec;
    % heading of shadow vehicle
    psi_s = s_pose(3);
    R = [cos(psi_s), -sin(psi_s); sin(psi_s), cos(psi_s)];
    Ri = R';
    
    % rotate diff vec around shadow vehicle
    dist_vec = Ri*diff_vec;
    
    % get cross track error as y coordinate of dist_vec multiplied by -1
    cross_track = dist_vec(2);

== matlab function LateralControlTutorial/Vehicle and Environment/Pack Ego Actor ==
  data: pose input; egoActor output Bus: BusActorsActors size=1; dx input; dy input; yawRate input
function egoActor = packEgo(pose,dx,dy,yawRate)
% Pack ego information into a single ego actor bus
%
% Imoprtant note:
% Output is a bus of type BusActorsActors. This is the same bus used by the
% Scenario Reader to output an individual actor. If you change the
% output bus name of Scenario Reader, change the output bus name here
% as well by clicking on 'Edit Data' in the menu above.

egoActor = struct(...
    'ActorID', 1,...
    'Position', [pose(1) pose(2) 0], ...
    'Velocity', [dx dy 0], ...
    'Roll', 0, ...
    'Pitch', 0, ...
    'Yaw', pose(3), ...
    'AngularVelocity', [0 0 yawRate]);

== matlab function LateralControlTutorial/Stanley Controller/MATLAB Function ==
  data: e_psi input; delta output; e_y input; v input; rho input; r input; steerDiff input
function delta = fcn(e_psi, e_y, v, rho, r, steerDiff)
m = 2000;
lf = 1.4;
lr = 1.6;
cf = 12e3;

r_traj = v.^2*rho;

e_psi_ss = (m*v*r_traj)/cf/(1+lr/lf);

k = 700;
k_soft = 1;
k_d_yaw = .1;
k_d_steer = .05;

delta = -(e_psi-e_psi_ss)+atan2(k*e_y,k_soft+v)+k_d_yaw*(r_traj-r)+k_d_steer*steerDiff;

== matlab function LateralControlTutorial/Vehicle and Environment/MATLAB Function2 ==
  data: v_pose input; cross_track output; s_pose input
function cross_track = cross_track_calc(v_pose, s_pose)
    v_vec = [v_pose(1); v_pose(2)];
    s_vec = [s_pose(1); s_pose(2)];
    % vector pointing from shadow vehicle to real vehicle
    diff_vec = v_vec - s_vec;
    % heading of shadow vehicle
    psi_s = s_pose(3);
    R = [cos(psi_s), -sin(psi_s); sin(psi_s), cos(psi_s)];
    Ri = R';
    
    % rotate diff vec around shadow vehicle
    dist_vec = Ri*diff_vec;
    
    % get cross track error as y coordinate of dist_vec multiplied by -1
    cross_track = dist_vec(2);

== matlab function LateralControlTutorial/Basic Lateral Controller1/Error Metric ==
  data: currPose input size=[1 3]; refPose input size=[1 3]; lateralError output; wheelbase parameter; headingError output; clock input
function [lateralError, headingError] = fcn(currPose, refPose, wheelbase, clock)

%   Copyright 2018 The MathWorks, Inc.

currPose(:,3) = deg2rad(currPose(:,3));
refPose(:,3)  = deg2rad(refPose(:,3));

%Convert current pose to front wheel coordinate
currPoseF = coder.nullcopy(zeros(1, 3));

currPoseF = driving.internal.control.rearPoseToFrontPose(currPose, wheelbase);

lateralError = sign(refPose(2) - currPoseF(2))*norm(currPoseF(1:2) - refPose(1:2));

headingError = rad2deg(currPose(:, 3) - refPose(:,3));

== matlab function LateralControlTutorial/Basic Lateral Controller1/MATLAB Function1 ==
  data: v_pose input; cross_track output; s_pose input
function cross_track = cross_track_calc(v_pose, s_pose)
    v_vec = [v_pose(1); v_pose(2)];
    s_vec = [s_pose(1); s_pose(2)];
    % vector pointing from shadow vehicle to real vehicle
    diff_vec = v_vec - s_vec;
    % heading of shadow vehicle
    psi_s = s_pose(3);
    R = [cos(psi_s), -sin(psi_s); sin(psi_s), cos(psi_s)];
    Ri = R';
    
    % rotate diff vec around shadow vehicle
    dist_vec = Ri*diff_vec;
    
    % get cross track error as y coordinate of dist_vec multiplied by -1
    cross_track = dist_vec(2);
